simulink model "tutorial_simulink_6"  (R2024b)
settings: Solver=VariableStepAuto  StartTime=0.0  StopTime=15.0  RelTol=1e-3
undefined symbols (not defined in the file): b, k, m, v0, x0
settings Model: Creator=俞书阳  LastModifiedBy=user

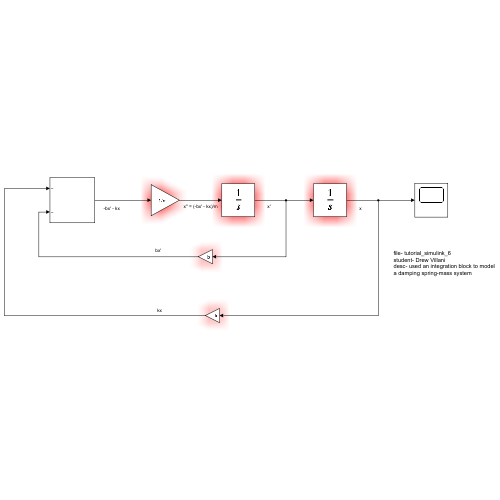
[thumbnail: Simulink's stored preview of the top-level diagram]
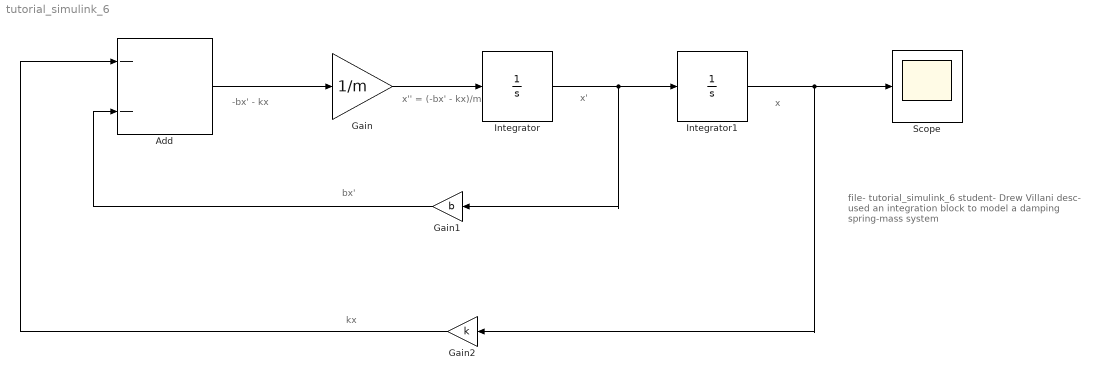
== system tutorial_simulink_6 ==
  note: file- tutorial_simulink_6
      | student- Drew Villani
      | desc- used an integration block to model
      | a damping spring-mass system
  note: kx
  note: bx'
  note: x'
  note: -bx' - kx
  note: x'' = (-bx' - kx)/m
  note: x
  Add : Sum  Inputs=--
  Gain : Gain  Gain=1/m
  Gain1 : Gain  Gain=b
  Gain2 : Gain  Gain=k
  Integrator : Integrator  InitialCondition=v0
  Integrator1 : Integrator  InitialCondition=x0
  Scope : Scope
  wires:
  Add/1 -> Gain/1
  Gain/1 -> Integrator/1
  Integrator/1 -> Gain1/1, Integrator1/1
  Integrator1/1 -> Gain2/1, Scope/1
  Gain1/1 -> Add/2
  Gain2/1 -> Add/1
